simulink model "example_main_NDI_f16"  (R2020a)
settings: Solver=ode4  StartTime=0.0  StopTime=75  FixedStep=0.01  RelTol=1e-3
PreLoadFcn:
  | PreLoadFcn
values from neighbouring files (symbols this model uses):
  g = 32.17    [PreLoadFcn.m]
  N = [ 1      0     0.25 ... (first row only)    [PreLoadFcn.m]
  state0 = [IC.npos IC.epos IC.alt IC.q0 IC.q1 IC.q2 IC.q3  IC.p IC.q IC.r IC.alpha IC.beta IC.mu IC.Vt IC.chi IC.gamma]    [PreLoadFcn.m]
undefined symbols (not defined in the file or in its folder): Aactuator, ac, AeroCoeff, EngineTable, ft, IC, kg, m, Newton, PIController, Raphson, s, sigbuilder_block, slug
libraries: aerolibconvert2 x19, simulink x13, sharedutil x1
(part 3 of 6)

== system example_main_NDI_f16/F-16 Vehicle Systems Model/Vehicle/Actuators (no roll off)1 ==
  note: 這種建模方式會得到跟順淵不同的結果
  Command : Inport
  "Mach " : Inport  Port=2
  alt : Inport  Port=3
  alpha,beta : Inport  Port=4
  Aileron Saturation : Saturate  UpperLimit=21.5  LowerLimit=-21.5
  Demux1 : Demux  Outputs=6
  Elevator Saturation : Saturate  UpperLimit=25  LowerLimit=-25
  Engine block : Subsystem
  Fcn : Fcn  Expr=u(1)*cos(u(2))*cos(u(3))
  Integrator (degrees) : Integrator  Commented=through  InitialCondition=0.015206  UpperSaturationLimit=30  LowerSaturationLimit=-30
  Integrator (degrees)1 : Integrator  Commented=through  UpperSaturationLimit=30  LowerSaturationLimit=-30
  Integrator (degrees)2 : Integrator  Commented=on  UpperSaturationLimit=30  LowerSaturationLimit=-30
  Integrator(degrees) : Integrator  Commented=on  InitialCondition=-0.051516  UpperSaturationLimit=21.5  LowerSaturationLimit=-21.5
  "Integrator(degrees) " : Integrator  Commented=on  InitialCondition=-4.2454  UpperSaturationLimit=25  LowerSaturationLimit=-25
  Mux1 : Mux  Inputs=2
  Mux9 : Mux  Inputs=6
  Rate Limiter : RateLimiter  RisingSlewLimit=+60  FallingSlewLimit=-60  SampleTimeMode=inherited
  Rate Limiter1 : RateLimiter  RisingSlewLimit=+80  FallingSlewLimit=-80  SampleTimeMode=inherited
  Rate Limiter2 : RateLimiter  RisingSlewLimit=+120  FallingSlewLimit=-120  SampleTimeMode=inherited
  Rate Limiter3 : RateLimiter  RisingSlewLimit=+60  FallingSlewLimit=-60  SampleTimeMode=inherited
  Rate Limiter4 : RateLimiter  RisingSlewLimit=+60  FallingSlewLimit=-60  SampleTimeMode=inherited
  Rudder Saturation : Saturate  UpperLimit=30  LowerLimit=-30
  Saturation : Saturate  UpperLimit=50000  LowerLimit=0
  Saturation Dynamic : simulink/Discontinuities/Saturation Dynamic  OutMin=[]  OutMax=[]  OutDataTypeStr=Inherit: Same as second input  OutDataType=fixdt(1, 16)  OutScaling=2^-10  DoSatur=off
  TVC_Y Saturation : Saturate  UpperLimit=15  LowerLimit=-15
  TVC_Z Saturation : Saturate  UpperLimit=15  LowerLimit=-15
  Transfer Fcn{,1..4} (5 alike) : TransferFcn  Numerator=[20.202]  Denominator=[1 20.202]
  r2d2 : Gain  Gain=-1  SaturateOnIntegerOverflow=on  OutDataTypeStr=Inherit: Same as input  ParamDataTypeStr=Inherit: Same as input
  Actuator : Outport  VectorParamsAs1DForOutWhenUnconnected=off
  wires:
  Mux9/1 -> Actuator/1
  Command/1 -> Demux1/1
  Transfer Fcn/1 -> Mux9/2  "elevator"
  Transfer Fcn1/1 -> Mux9/3  "Aileron"
  Transfer Fcn2/1 -> Mux9/4  "Rudder"
  Saturation Dynamic/1 -> Mux9/1  "thrust"
  Transfer Fcn4/1 -> Mux9/6  "yaw vector"
  Transfer Fcn3/1 -> Mux9/5  "pitch vector"
  r2d2/1 -> Saturation/1
  alt/1 -> r2d2/1
  Demux1/1 -> Saturation Dynamic/2
  "Mach "/1 -> Mux1/1
  alpha,beta/1 -> Mux1/2
  Mux1/1 -> Fcn/1
  Fcn/1 -> Engine block/1(Mach)
  Saturation/1 -> Engine block/2(Attitude)
  Engine block/2(T_min) -> Saturation Dynamic/3
  Engine block/1(T_max) -> Saturation Dynamic/1
  Demux1/2 -> Elevator Saturation/1
  Elevator Saturation/1 -> Rate Limiter/1
  Demux1/3 -> Aileron Saturation/1
  Aileron Saturation/1 -> Rate Limiter1/1
  Demux1/4 -> Rudder Saturation/1
  Rudder Saturation/1 -> Rate Limiter2/1
  Demux1/5 -> TVC_Z Saturation/1
  TVC_Z Saturation/1 -> Rate Limiter3/1
  Demux1/6 -> TVC_Y Saturation/1
  TVC_Y Saturation/1 -> Rate Limiter4/1
  Rate Limiter/1 -> Transfer Fcn/1
  Rate Limiter1/1 -> Transfer Fcn1/1
  Rate Limiter2/1 -> Transfer Fcn2/1
  Rate Limiter3/1 -> Transfer Fcn3/1
  Rate Limiter4/1 -> Transfer Fcn4/1

== system example_main_NDI_f16/F-16 Vehicle Systems Model/Vehicle/Aerodynamics ==
  note: TODO: 這全部源自PlantData(物理系統)，不用感測器
  note: TODO: 這攻角、速度 來自感測器、AeroData System
  note: X
      | Y
      | Z
      | L
      | M
      | N
  note: 攻角 $\alpha$ 限制 -20 ~ 90度
      | 側滑角 $\beta$ 限制 -30 ~ 30 度
      | 馬赫數限制 0.1 ~ 0.6 度
  In Bus Element7 : Inport  PortName=EnvData  Element=P
  In Bus Element8 : Inport  PortName=EnvData  Element=AirDensity
  In Bus Element9 : Inport  PortName=EnvData  Element=qbar
  fcs_cmd : Inport  Port=2
  " SB (deg)" : Inport  Port=3
  In Bus Element : Inport  Port=4  PortName=PlantData  Element=p
  In Bus Element1 : Inport  Port=4  PortName=PlantData  Element=q
  In Bus Element2 : Inport  Port=4  PortName=PlantData  Element=r
  In Bus Element3 : Inport  Port=4  PortName=PlantData  Element=alpha
  In Bus Element10 : Inport  Port=4  PortName=PlantData  Element=alpha
  In Bus Element4 : Inport  Port=4  PortName=PlantData  Element=beta
  In Bus Element6 : Inport  Port=4  PortName=PlantData  Element=Vt
  In Bus Element5 : Inport  Port=4  PortName=PlantData  Element=Vt
  Aerofynamic Coefficients : Subsystem
  AirframeActuators (no roll off) : Subsystem
  Angle Conversion1 : aerolibconvert2/Angle Conversion  IU=rad  OU=deg
  Angle Conversion2 : aerolibconvert2/Angle Conversion  IU=rad  OU=deg
  Angle Conversion3 : aerolibconvert2/Angle Conversion  IU=rad  OU=deg
  Bus Creator : BusCreator  Inputs=4
  Bus Selector : BusSelector  OutputSignals=Elevator_deg,Aileron_deg,Rudder_deg
  Bus Selector1 : BusSelector  OutputSignals=Aileron_deg,Rudder_deg,Elevator_deg
  Bus Selector2 : BusSelector  OutputSignals=LEF_deg
  Cbar(ft)1 : Constant  Value=ac.cbar
  Ground : Ground
  Leading Edge Flap : Subsystem
  Mux1 : Mux  Inputs=3
  Mux2 : Mux
  Product{6,9..14} (7 alike) : Product
  Sref(ft^2) : Constant  Value=ac.S
  Velocity Conversion : aerolibconvert2/Velocity Conversion  IU=ft/s  OU=m/s
  b(ft)1 : Constant  Value=ac.b
  FM : Outport
  Bus Element Out : Outport  Port=2  PortName=ActSensor_Out
  wires:
  Bus Selector/2 -> Aerofynamic Coefficients/5(alieron (deg))  "<Aileron_deg>"
  " SB (deg)"/1 -> Aerofynamic Coefficients/7(SB (deg))
  In Bus Element1/1 -> Aerofynamic Coefficients/10(q)
  In Bus Element/1 -> Aerofynamic Coefficients/9(p)
  Bus Selector/3 -> Aerofynamic Coefficients/6(rudder (deg))  "<Rudder_deg>"
  Angle Conversion2/1 -> Aerofynamic Coefficients/2(beta (deg))
  Angle Conversion1/1 -> Aerofynamic Coefficients/1(alpha (deg))
  In Bus Element2/1 -> Aerofynamic Coefficients/11(r)
  [LEF_deg] -> Aerofynamic Coefficients/3(LEF (deg))
  Bus Selector/1 -> Aerofynamic Coefficients/4(elevator (deg))  "<Elevator_deg>"
  Ground/1 -> Aerofynamic Coefficients/13(h_AGL), Aerofynamic Coefficients/12(GearAngle)
  Mux1/1 -> Product9/2
  [qbar_S] -> Product9/1
  Aerofynamic Coefficients/6(Cn_T) -> Product14/2
  Aerofynamic Coefficients/5(Cm_T) -> Product12/2
  [qbar_S_cbar] -> Product12/1  "qbar_S_cbar"
  Aerofynamic Coefficients/4(Cl_T) -> Product13/2
  [qbar_S_b] -> Product13/1, Product14/1  "qbar_S_b"
  Aerofynamic Coefficients/1(CX_T) -> Mux1/1
  Aerofynamic Coefficients/2(CY_T) -> Mux1/2
  Aerofynamic Coefficients/3(CZ_T) -> Mux1/3
  Product13/1 -> Mux2/2
  Product12/1 -> Mux2/3
  Product14/1 -> Mux2/4
  Product9/1 -> Mux2/1
  Mux2/1 -> FM/1
  Sref(ft^2)/1 -> Product6/2
  b(ft)1/1 -> Product11/2  "b"
  Product11/1 -> [qbar_S_b]
  Product10/1 -> [qbar_S_cbar]
  Cbar(ft)1/1 -> Product10/2  "cbar"
  In Bus Element9/1 -> Product6/1  "qbar"
  Product6/1 -> Product11/1, Product10/1, [qbar_S]  "qbar_S"
  Leading Edge Flap/2(ActPositions) -> [LEF_deg]
  Velocity Conversion/1 -> Leading Edge Flap/1(vt (m/s))  "vt (m/s)"
  In Bus Element6/1 -> Aerofynamic Coefficients/8(vt (ft/s))
  In Bus Element8/1 -> Leading Edge Flap/2(rho (kg/m^3))
  In Bus Element7/1 -> Leading Edge Flap/3(P (Pa))
  AirframeActuators (no roll off)/1(ActPositions) -> Bus Selector/1
  fcs_cmd/1 -> AirframeActuators (no roll off)/1(fcs_cmd)
  In Bus Element3/1 -> Angle Conversion1/1
  In Bus Element4/1 -> Angle Conversion2/1
  In Bus Element5/1 -> Velocity Conversion/1  "vt (ft/s)"
  AirframeActuators (no roll off)/2(ActSensor_Out) -> Bus Selector1/1
  Bus Selector1/1 -> Bus Creator/1  "<Aileron_deg>"
  Bus Selector1/2 -> Bus Creator/2  "<Rudder_deg>"
  Bus Selector1/3 -> Bus Creator/3  "<Elevator_deg>"
  Bus Creator/1 -> Bus Element Out/1
  In Bus Element10/1 -> Angle Conversion3/1
  Angle Conversion3/1 -> Leading Edge Flap/4(alpha (deg))
  Leading Edge Flap/1(ActSensor_Out) -> Bus Selector2/1
  Bus Selector2/1 -> Bus Creator/4  "<LEF_deg>"

== system example_main_NDI_f16/F-16 Vehicle Systems Model/Vehicle/Propulsion ==
  note: 高度限制 0 ~ 50000 ft
      | 馬赫數限制 0 ~ 1 馬赫
  note: Thrust Vector Nozzle Module 向量噴嘴模組
  note: Commands_TVC_Z_pitch
      | Commands_TVC_Y_yaw
  note: Inlet 進氣道
  In Bus Element1 : Inport  PortName=EnvData  Element=Mach
  Bus Element In2 : Inport  Port=2  PortName=fadec_cmd
  In Bus Element2 : Inport  Port=2  PortName=fadec_cmd  Element=thrust
  Bus Element In1 : Inport  Port=3  PortName=PlantData  Element=beta
  Bus Element In : Inport  Port=3  PortName=PlantData  Element=alpha
  In Bus Element : Inport  Port=3  PortName=PlantData  Element=altitude
  Actuators : Subsystem
  Afterburning Turbofan Jet Engine : Subsystem
  Cos : Trigonometry  Operator=cos
  Cos1 : Trigonometry  Operator=cos
  Product : Product  Inputs=3
  Saturation Dynamic : simulink/Discontinuities/Saturation Dynamic  OutMin=[]  OutMax=[]  OutDataTypeStr=Inherit: Same as second input  OutDataType=fixdt(1, 16)  OutScaling=2^-10  DoSatur=off
  Thrust Vector Nozzle ZY : Subsystem
  nozzle position : Constant  Value=ac.lt
  r2d1 : Gain  Gain=-1  SaturateOnIntegerOverflow=on  OutDataTypeStr=Inherit: Same as input  ParamDataTypeStr=Inherit: Same as input
  FM : Outport
  Bus Element Out : Outport  Port=2  PortName=ActSensor_Out
  Bus Element Out1 : Outport  Port=3  PortName=PropData  Element=Tx
  Bus Element Out2 : Outport  Port=3  PortName=PropData  Element=Ty
  Bus Element Out3 : Outport  Port=3  PortName=PropData  Element=Tz
  Bus Element Out4 : Outport  Port=3  PortName=PropData  Element=T
  wires:
  Actuators/2(ActSensor_Out) -> Bus Element Out/1
  nozzle position/1 -> Thrust Vector Nozzle ZY/3(" lt")
  Actuators/1(ActPositions) -> Thrust Vector Nozzle ZY/2(Actuator (deg))
  Thrust Vector Nozzle ZY/1(FM) -> FM/1
  Product/1 -> Afterburning Turbofan Jet Engine/1(Mach)
  r2d1/1 -> Afterburning Turbofan Jet Engine/2(H (ft))
  Cos/1 -> Product/2
  Saturation Dynamic/1 -> Bus Element Out4/1, Thrust Vector Nozzle ZY/1(T)  "Thrust (lbf)"
  Bus Element In1/1 -> Cos1/1  "beta (rad)"
  Afterburning Turbofan Jet Engine/2(T_min) -> Saturation Dynamic/3
  In Bus Element1/1 -> Product/1
  Cos1/1 -> Product/3
  Bus Element In/1 -> Cos/1  "alpha (rad)"
  Afterburning Turbofan Jet Engine/1(T_max) -> Saturation Dynamic/1
  In Bus Element/1 -> r2d1/1
  In Bus Element2/1 -> Saturation Dynamic/2  "Commands_Tc"
  Bus Element In2/1 -> Actuators/1(Commands)
  Thrust Vector Nozzle ZY/2(Tx) -> Bus Element Out1/1
  Thrust Vector Nozzle ZY/3(Ty) -> Bus Element Out2/1
  Thrust Vector Nozzle ZY/4(Tz) -> Bus Element Out3/1

== system example_main_NDI_f16/F-16 Vehicle Systems Model/pqr NDI Controller/TVC OFF ==
  note: 【無向量噴嘴控制】
      | (註：有/無向量噴嘴的差異之處在於 "粉紅色模塊" 的內容)
  note: 沒有控制配置，也不需要，
      | 因為沒有多餘的控制面可用
  note: gp_da1
      | gp_da2
      | gp_dr1
      | gp_dr2
      | m_de
      | gr_da1
      | gr_da2
      | gr_dr1
      | gr_dr2
  note: $\hat{L}, \hat{M}, \hat{N}$
  coef M : Inport
  control g : Inport  Port=2
  pqr dot desire : Inport  Port=3
  In Bus Element : Inport  Port=4  PortName=PlantData  Element=PropBus.T
  p q r : Inport  Port=5
  In Bus Element2 : Inport  Port=6  PortName=AirData  Element=alpha
  In Bus Element1 : Inport  Port=6  PortName=AirData  Element=Vt
  " f1" : MATLAB Function  TreatAsAtomicUnit=on
  Constant : Constant  Value=0
  Constant1 : Constant  Value=0
  Ix(slug*ft^2)1 : Constant  Value=ac.Ix
  Ixz(slug*ft^2)1 : Constant  Value=ac.Ixz
  Iy(slug*ft^2)1 : Constant  Value=ac.Iy
  Iz(slug*ft^2)1 : Constant  Value=ac.Iz
  Sum : Sum  Inputs=+-|
  Terminator : Terminator
  Terminator1 : Terminator
  control matrix g1 : Subsystem
  innear NDI : MATLAB Function  TreatAsAtomicUnit=on
  TVC_z : Outport  VectorParamsAs1DForOutWhenUnconnected=off
  "TVC_y " : Outport  Port=2  VectorParamsAs1DForOutWhenUnconnected=off
  elevator : Outport  Port=3  VectorParamsAs1DForOutWhenUnconnected=off
  aileron : Outport  Port=4  VectorParamsAs1DForOutWhenUnconnected=off
  rudder : Outport  Port=5  VectorParamsAs1DForOutWhenUnconnected=off
  wires:
  Iy(slug*ft^2)1/1 -> " f1"/4(Iy)
  Ixz(slug*ft^2)1/1 -> " f1"/6(Ixz)
  Iz(slug*ft^2)1/1 -> " f1"/5(Iz)
  pqr dot desire/1 -> Sum/1
  Sum/1 -> innear NDI/1(y_bar)
  p q r/1 -> " f1"/2(pqr)
  Ix(slug*ft^2)1/1 -> " f1"/3(Ix)
  " f1"/1(f) -> Sum/2
  Constant1/1 -> "TVC_y "/1
  control matrix g1/1(g_1 Row1) -> innear NDI/2(g_row1)
  innear NDI/3(rudder) -> rudder/1
  control matrix g1/3(g_1 Row3) -> innear NDI/4(g_row3)
  innear NDI/2(elevator) -> elevator/1
  control g/1 -> control matrix g1/1(coef g)
  In Bus Element/1 -> control matrix g1/2(Thrust T)
  innear NDI/1(aileron) -> aileron/1
  control matrix g1/2(g_1 Row2) -> innear NDI/3(g_row2)
  coef M/1 -> " f1"/1(moments)
  Constant/1 -> TVC_z/1
  In Bus Element1/1 -> Terminator/1
  In Bus Element2/1 -> Terminator1/1

== system example_main_NDI_f16/F-16 Vehicle Systems Model/pqr NDI Controller/TVC ON ==
  note: $\hat{L}, \hat{M}, \hat{N}$
  note: TODO:
      | 1. 控制配置的權重矩陣 參數化、拿出來外面、放進PreLoadFcn.m
      | 2. 改成Variant Subsystem
  note: 控制配置：
      | 1. 菊鍊式
      | 2. 聯動式
  note: gp_da1
      | gp_da2
      | gp_dr1
      | gp_dr2
      | m_de
      | gr_da1
      | gr_da2
      | gr_dr1
      | gr_dr2
  note: 【有向量噴嘴控制】
      | (註：有/無向量噴嘴的差異之處在於 "粉紅色模塊" 的內容)
  coef M : Inport
  control g : Inport  Port=2
  pqr dot desire : Inport  Port=3
  In Bus Element : Inport  Port=4  PortName=PlantData  Element=PropBus.T
  In Bus Element2 : Inport  Port=5  PortName=AirData  Element=alpha
  In Bus Element1 : Inport  Port=5  PortName=AirData  Element=Vt
  p q r : Inport  Port=6
  " f1" : MATLAB Function  TreatAsAtomicUnit=on
  Control Allocation : MATLAB Function  TreatAsAtomicUnit=on
  Ix(slug*ft^2)1 : Constant  Value=ac.Ix
  Ixz(slug*ft^2)1 : Constant  Value=ac.Ixz
  Iy(slug*ft^2)1 : Constant  Value=ac.Iy
  Iz(slug*ft^2)1 : Constant  Value=ac.Iz
  Sum : Sum  Inputs=+-|
  control matrix g1 : Subsystem
  weighting matrix N : Constant  Value=N
  TVC_z : Outport  VectorParamsAs1DForOutWhenUnconnected=off
  "TVC_y " : Outport  Port=2  VectorParamsAs1DForOutWhenUnconnected=off
  elevator : Outport  Port=3  VectorParamsAs1DForOutWhenUnconnected=off
  aileron : Outport  Port=4  VectorParamsAs1DForOutWhenUnconnected=off
  rudder : Outport  Port=5  VectorParamsAs1DForOutWhenUnconnected=off
  wires:
  coef M/1 -> " f1"/1(moments)
  p q r/1 -> " f1"/2(pqr)
  " f1"/1(f) -> Sum/2
  Sum/1 -> Control Allocation/1(y_bar)
  pqr dot desire/1 -> Sum/1
  In Bus Element/1 -> control matrix g1/2(Thrust T)
  control g/1 -> control matrix g1/1(coef g)
  control matrix g1/1(g_1 Row1) -> Control Allocation/2(g_row1)
  control matrix g1/2(g_1 Row2) -> Control Allocation/3(g_row2)
  control matrix g1/3(g_1 Row3) -> Control Allocation/4(g_row3)
  Control Allocation/3(rudder) -> rudder/1
  Control Allocation/2(elevator) -> elevator/1
  Control Allocation/1(aileron) -> aileron/1
  Control Allocation/4(TVC_y) -> "TVC_y "/1
  Control Allocation/5(TVC_z) -> TVC_z/1
  In Bus Element2/1 -> Control Allocation/6(alpha)
  Iy(slug*ft^2)1/1 -> " f1"/4(Iy)
  Ix(slug*ft^2)1/1 -> " f1"/3(Ix)
  Iz(slug*ft^2)1/1 -> " f1"/5(Iz)
  Ixz(slug*ft^2)1/1 -> " f1"/6(Ixz)
  weighting matrix N/1 -> Control Allocation/7(N)
  In Bus Element1/1 -> Control Allocation/5(Vt)

== system example_main_NDI_f16/F-16 Vehicle Systems Model/μαβ NDI Controller/command matrix (5.5.4) ==
  note: $g_2 {\left(x\right)}={\left[\begin{array}{ccc} g_{\mu_p } & g_{\mu_q } & g_{\mu_r } \\ g_{\alpha_p } & g_{\alpha_q } & g_{\alpha_r } \\ g_{\beta_p } & g_{\beta_q } & g_{\beta_r } \end{array}\right]}={\left[\begin{array}{ccc} \mathrm{cos}\alpha \mathrm{sec}\beta & 0 & \mathrm{sin}\alpha \mathrm{sec}\beta \\ -\mathrm{cos}\alpha \mathrm{tan}\beta & 1 & -\mathrm{sin}\alpha \mathrm{tan}\beta \\ \mathrm{sin}\alpha & 0 & -\mathrm{cos}\alpha \end{array}\right]}$
  α : Inport
  β : Inport  Port=2
  (1,1) : Fcn  Expr=1/cos(u(2)) * cos(u(1))
  (1,2) : Constant  Value=0
  (1,3) : Fcn  Expr=1/cos(u(2)) * sin(u(1))
  (2,1) : Fcn  Expr=-tan(u(2)) * cos(u(1))
  (2,2) : Constant
  (2,3) : Fcn  Expr=-tan(u(2)) * sin(u(1))
  (3,1) : Fcn  Expr=sin(u(1))
  (3,2) : Constant  Value=0
  (3,3) : Fcn  Expr=-cos(u(1))
  Create 3x3 Matrix : sharedutil/Create 3x3 Matrix  aMode=aMode
      settings: SourceProductBaseCode=AE,PW,MT,VE,VP
  Mux4 : Mux  Inputs=2
  g2 : Outport  VectorParamsAs1DForOutWhenUnconnected=off
  wires:
  α/1 -> Mux4/1
  β/1 -> Mux4/2
  Mux4/1 -> (3,3)/1, (3,1)/1, (2,3)/1, (1,1)/1, (1,3)/1, (2,1)/1
  Create 3x3 Matrix/1 -> g2/1
  (2,2)/1 -> Create 3x3 Matrix/5
  (2,1)/1 -> Create 3x3 Matrix/4
  (2,3)/1 -> Create 3x3 Matrix/6
  (1,3)/1 -> Create 3x3 Matrix/3
  (3,1)/1 -> Create 3x3 Matrix/7
  (1,2)/1 -> Create 3x3 Matrix/2
  (3,2)/1 -> Create 3x3 Matrix/8
  (1,1)/1 -> Create 3x3 Matrix/1
  (3,3)/1 -> Create 3x3 Matrix/9

== system example_main_NDI_f16/F-16 Vehicle Systems Model/μαβ NDI Controller/f2 (5.5.3) ==
  note: 有指定port dimensions=3。
      | 否則，雖然可以正常執行程式，
      | 但是t=0會跳出錯誤訊息說下一模塊"attitude NDI"內的矩陣運算的dimensions不一致
  note: mu alpha beta
  note: 11 gravity
  note: 10 T
  note: 9 mass
  note: 8 L
  note: 7 Y
  note: 6 D
  note: 1 Vt alpha beta mu gamma
  note: 11 gravity
  note: 9 mass
  note: 6 Xbar Ybar Zbar
  note: 1 Vinf alpha beta mu gamma
  note: 10 T
  aero V : Inport
  X,Y,Z : Inport  Port=2
  gravity : Inport  Port=3
  Thrust : Inport  Port=4
  Add : Sum  Inputs=+++
  Drag : Fcn  Expr=-u(6)*cos(u(2))*cos(u(3))-u(7)*sin( u(3) )-u(8)*sin(u(2))*cos(u(3))
  Lift : Fcn  Expr=u(6)*sin(u(2))-u(8)*cos(u(2))
  Mux : Mux  Inputs=3
  Mux1 : Mux  Inputs=7
  Mux2 : Mux  Inputs=2
  Side Force : Fcn  Expr=-u(6)*cos(u(2))*sin(u(3))+u(7)*cos( u(3) )-u(8)*sin(u(2))*sin(u(3))
  f_alpha : Fcn  Expr=( -u(8)+u(9)*u(11)*cos(u(5))*cos(u(4))-u(10)*sin(u(2)) ) / ( u(9)*u(1)*cos(u(3)) )
  f_beta : Fcn  Expr=( u(7)*cos(u(3))+u(9)*u(11)*cos(u(5))*sin(u(4))-u(10)*cos(u(2))*sin(u(3)) ) / ( u(9)*u(1) )
  f_mu1 : Fcn  Expr=u(8)*( tan(u(5))*sin(u(4))+tan(u(3)) ) / ( u(9)*u(1) )
  f_mu2 : Fcn  Expr=(u(7)*tan(u(5))*cos(u(4))*cos(u(3)) -u(9)*u(11)*cos(u(5))*cos(u(4))*tan(u(3)) ) / ( u(9)*u(1) )
  f_mu3 : Fcn  Expr=u(10)*( sin(u(2))*tan(u(5))*sin(u(4)) + sin(u(2))*tan(u(3)) - cos(u(2))*tan(u(5))*cos(u(4))*sin(u(3)) ) / ( u(9)*u(1) )
  m(slugs) : Constant  Value=ac.m
  f2 : Outport  PortDimensions=3  VectorParamsAs1DForOutWhenUnconnected=off
  D : Outport  Port=2  VectorParamsAs1DForOutWhenUnconnected=off
  Y : Outport  Port=3  VectorParamsAs1DForOutWhenUnconnected=off
  L : Outport  Port=4  VectorParamsAs1DForOutWhenUnconnected=off
  wires:
  Mux/1 -> f2/1
  f_beta/1 -> Mux/3
  aero V/1 -> Mux1/1, Mux2/1  "Vt, α, β, μ, γ"
  X,Y,Z/1 -> Mux2/2  "Xbar, Ybar, Zbar"
  Mux2/1 -> Lift/1, Drag/1, Side Force/1
  Mux1/1 -> f_alpha/1, f_beta/1, f_mu2/1, f_mu1/1, f_mu3/1
  Drag/1 -> Mux1/2, D/1  "D"
  Side Force/1 -> Mux1/3, Y/1  "Y"
  Lift/1 -> Mux1/4, L/1  "L"
  m(slugs)/1 -> Mux1/5
  Thrust/1 -> Mux1/6  "T"
  gravity/1 -> Mux1/7  "g"
  f_alpha/1 -> Mux/2
  f_mu2/1 -> Add/2
  f_mu1/1 -> Add/1
  Add/1 -> Mux/1
  f_mu3/1 -> Add/3

== system example_main_NDI_f16/F-16 Vehicle Systems Model/Aerodynamic1/NDI Aerofynamic Coefficients/CXT ==
  note: 氣動力表格僅提供到攻角到
      | 45度，超過45度後皆採用45
      | 度的氣動力係數
  note: $\Delta C_{X_{LEF} } =C_{X_{LEF} } {\left(\alpha ,\beta \right)}-C_X {\left(\alpha ,\beta ,\delta_e =0°\right)}$
  note: $C_{X,T} =C_X {\left(\alpha ,\beta ,\delta_e \right)}+\Delta C_{X_{LEF} } ∙{\left(1-\frac{\delta_{LEF} }{25°}\right)}+\frac{q\bar{c} }{2V_T }∙{\left[C_{X_q } {\left(\alpha \right)}+\Delta C_{X_{q_{LEF} } } {\left(\alpha \right)}∙{\left(1-\frac{\delta_{LEF} }{25°}\right)}\right]}+\Delta C_{X_{SB} } {\left(\alpha \right)}∙{\left(\frac{\delta_{SB} }{60°}\right)}$
  note: 體軸 x 方向之氣動力係數 (total x-axis force coefficient)：
  alpha (deg) : Inport
  beta (deg) : Inport  Port=2
  elevator (deg) : Inport  Port=3
  dlef : Inport  Port=4
  qc_2v : Inport  Port=5
  sb : Inport  Port=6
  Add : Sum  Inputs=+-
  Add1 : Sum  Inputs=++++
  Add2 : Sum
  Cx : Interpolation_n-D  NumberOfTableDimensions=3  Table=AeroCoeff.Cx
      settings: InputPortMap=u0,u1,u2,u3,u4,u5
  Cx_elevator0 : Interpolation_n-D  Table=AeroCoeff.Cx_elevator0
  Cx_lef : Interpolation_n-D  Table=AeroCoeff.Cx_lef
  Cx_q : Interpolation_n-D  NumberOfTableDimensions=1  Table=AeroCoeff.Cx_q
      settings: InputPortMap=u0,u1
  Cx_q_lef : Interpolation_n-D  NumberOfTableDimensions=1  Table=AeroCoeff.Cx_q_lef
      settings: InputPortMap=u0,u1
  Product{,1..3} (4 alike) : Product
  alpha Prelookup : PreLookup  BreakpointsData=AeroCoeff.alpha_prelookup  IndexSearchMethod=Linear search  BeginIndexSearchUsingPreviousIndexResult=on  DiagnosticForOutOfRangeInput=Warning
  beta Prelookup : PreLookup  BreakpointsData=AeroCoeff.beta_prelookup  IndexSearchMethod=Linear search  BeginIndexSearchUsingPreviousIndexResult=on  DiagnosticForOutOfRangeInput=Warning
  dCX_sb : Interpolation_n-D  NumberOfTableDimensions=1  Table=AeroCoeff.dCX_sb
      settings: InputPortMap=u0,u1
  elevator Prelookup : PreLookup  BreakpointsData=AeroCoeff.elevator_prelookup2  IndexSearchMethod=Linear search  BeginIndexSearchUsingPreviousIndexResult=on  DiagnosticForOutOfRangeInput=Warning
  Cx_tot : Outport  VectorParamsAs1DForOutWhenUnconnected=off
  wires:
  beta Prelookup/2 -> Cx_elevator0/4, Cx_lef/4, Cx/4
  alpha (deg)/1 -> alpha Prelookup/1
  beta Prelookup/1 -> Cx_elevator0/3, Cx_lef/3, Cx/3
  Cx_lef/1 -> Add/1
  alpha Prelookup/1 -> Cx_q_lef/1, dCX_sb/1, Cx_q/1, Cx_elevator0/1, Cx/1, Cx_lef/1
  elevator Prelookup/2 -> Cx/6
  elevator (deg)/1 -> elevator Prelookup/1
  beta (deg)/1 -> beta Prelookup/1
  Add/1 -> Product/1
  alpha Prelookup/2 -> Cx_q_lef/2, dCX_sb/2, Cx_q/2, Cx_elevator0/2, Cx_lef/2, Cx/2
  Product/1 -> Add1/2
  elevator Prelookup/1 -> Cx/5
  Add2/1 -> Product2/1
  Cx/1 -> Add1/1
  Cx_elevator0/1 -> Add/2
  Cx_q_lef/1 -> Product1/1
  Product1/1 -> Add2/2
  Cx_q/1 -> Add2/1
  dlef/1 -> Product/2, Product1/2
  Product2/1 -> Add1/3
  Add1/1 -> Cx_tot/1
  qc_2v/1 -> Product2/2
  dCX_sb/1 -> Product3/1
  sb/1 -> Product3/2
  Product3/1 -> Add1/4

== system example_main_NDI_f16/F-16 Vehicle Systems Model/Aerodynamic1/NDI Aerofynamic Coefficients/CYT ==
  note: 氣動力表格僅提供到攻角到
      | 45度，超過45度後皆採用45
      | 度的氣動力係數
  note: 氣動力表格僅提供到攻角到
      | 45度，超過45度後皆採用45
      | 度的氣動力係數
  note: 體軸 y 方向之氣動力係數 (total y-axis force coefficient)：
  note: $\Delta C_{Y_{LEF} }=C_{Y_{LEF} } {\left(\alpha ,\beta \right)}\ \ -C_Y {\left(\alpha ,\beta \right)}$
  note: $\Delta C_{Y_{\delta_r } }=C_{Y_{\delta_r =30°} } {\left(\alpha ,\beta \right)}-C_Y {\left(\alpha ,\beta \right)}$
  note: $C_{Y,T} =C_Y {\left(\alpha ,\beta \right)}+\Delta C_{Y_{LEF} } ∙{\left(1-\frac{\delta_{LEF} }{25°}\right)}+\frac{pb}{2V_T }∙{\left[C_{Y_p } {\left(\alpha \right)}+\Delta C_{{Y_p }_{LEF} } {\left(\alpha \right)}∙{\left(1-\frac{\delta_{LEF} }{25°}\right)}\right]}+\frac{rb}{2V_T }∙{\left[C_{Y_r } {\left(\alpha \right)}+\Delta C_{{Y_r }_{LEF} } {\left(\alpha \right)}∙{\left(1-\frac{\delta_{LEF} }{25°}\right)}\right]}+{\left[\Delta C_{Y_{\delta_a } } +\Delta C_{Y_{{\delta_a }_{LEF} } } ∙{\left(1-\frac{\delta_{LEF} }{25°}\right)}\right]}∙{\left(\frac{\delta_a }{20°}\right)}+\Delta C_{Y_{\delta_r } } ∙{\left(\frac{\delta_r }{30°}\right)}$
  note: $\Delta C_{Y_{{\delta_a }_{LEF} } } =C_{Y_{{\delta_a =20°}_{LEF} } } {\left(\alpha ,\beta \right)}-C_{Y_{LEF} } {\left(\alpha ,\beta \right)}-\Delta C_{Y_{\delta_a } }$
  note: $\Delta C_{Y_{\delta_a } }=C_{Y_{\delta_a =20°} } {\left(\alpha ,\beta \right)}-C_Y {\left(\alpha ,\beta \right)}$
  alpha (deg) : Inport
  beta (deg) : Inport  Port=2
  dlef : Inport  Port=3
  dail : Inport  Port=4
  drud : Inport  Port=5
  rb_2v : Inport  Port=6
  pb_2v : Inport  Port=7
  Add : Sum  Inputs=-+
  Add1 : Sum  Inputs=-+
  Add2 : Sum  Inputs=+--
  Add3 : Sum  Inputs=+-
  Add4 : Sum  Inputs=++++++
  Add5 : Sum
  Add6 : Sum
  Add7 : Sum
  Add8 : Sum  Inputs=++++
  CY : Interpolation_n-D  Table=AeroCoeff.CY
  CY_delta_ail : Interpolation_n-D  Table=AeroCoeff.CY_delta_ail
  CY_delta_ail_lef : Interpolation_n-D  Table=AeroCoeff.CY_delta_ail_lef
  CY_delta_r : Interpolation_n-D  Table=AeroCoeff.CY_delta_r
  CY_lef : Interpolation_n-D  Table=AeroCoeff.CY_lef
  CY_p : Interpolation_n-D  NumberOfTableDimensions=1  Table=AeroCoeff.CY_p
      settings: InputPortMap=u0,u1
  CY_r : Interpolation_n-D  NumberOfTableDimensions=1  Table=AeroCoeff.CY_r
      settings: InputPortMap=u0,u1
  Product{,1..7} (8 alike) : Product
  alpha Prelookup : PreLookup  BreakpointsData=AeroCoeff.alpha_prelookup  IndexSearchMethod=Linear search  BeginIndexSearchUsingPreviousIndexResult=on  DiagnosticForOutOfRangeInput=Warning
  beta Prelookup : PreLookup  BreakpointsData=AeroCoeff.beta_prelookup  IndexSearchMethod=Linear search  BeginIndexSearchUsingPreviousIndexResult=on  DiagnosticForOutOfRangeInput=Warning
  dCY_p_lef : Interpolation_n-D  NumberOfTableDimensions=1  Table=AeroCoeff.dCY_p_lef
      settings: InputPortMap=u0,u1
  dCY_r_lef : Interpolation_n-D  NumberOfTableDimensions=1  Table=AeroCoeff.dCY_r_lef
      settings: InputPortMap=u0,u1
  Cy_tot : Outport  VectorParamsAs1DForOutWhenUnconnected=off
  Cy_tot_n_mom : Outport  Port=2  VectorParamsAs1DForOutWhenUnconnected=off
  Cy_tot_n_da : Outport  Port=3  VectorParamsAs1DForOutWhenUnconnected=off
  Cy_tot_n_dr : Outport  Port=4  VectorParamsAs1DForOutWhenUnconnected=off
  wires:
  Add3/1 -> Cy_tot_n_dr/1, Product3/1
  beta Prelookup/2 -> CY_delta_r/4, CY_delta_ail_lef/4, CY_delta_ail/4, CY/4, CY_lef/4
  beta Prelookup/1 -> CY_delta_r/3, CY_delta_ail_lef/3, CY_delta_ail/3, CY/3, CY_lef/3
  Product7/1 -> Add4/6, Add8/4
  dlef/1 -> Product1/2, Product/2, Product4/2, Product6/1
  alpha Prelookup/1 -> dCY_p_lef/1, CY_p/1, dCY_r_lef/1, CY_r/1, CY_delta_r/1, CY_delta_ail_lef/1, CY_delta_ail/1, CY_lef/1, CY/1
  Add4/1 -> Cy_tot/1
  Add5/1 -> Cy_tot_n_da/1, Product2/1
  CY_p/1 -> Add7/1
  Add1/1 -> Add2/3, Add5/1
  CY_lef/1 -> Add/2, Add2/2
  Add/1 -> Product/1
  dCY_p_lef/1 -> Product6/2
  CY_delta_r/1 -> Add3/1
  CY_delta_ail_lef/1 -> Add2/1
  dCY_r_lef/1 -> Product4/1
  alpha (deg)/1 -> alpha Prelookup/1
  CY_r/1 -> Add6/1
  Product4/1 -> Add6/2
  Add2/1 -> Product1/1
  Product3/1 -> Add4/4
  CY/1 -> Add8/1, Add4/1, Add/1, Add1/1, Add3/2
  Product2/1 -> Add4/3
  Product/1 -> Add4/2, Add8/2
  alpha Prelookup/2 -> CY_p/2, dCY_p_lef/2, dCY_r_lef/2, CY_r/2, CY_delta_r/2, CY_delta_ail_lef/2, CY_delta_ail/2, CY_lef/2, CY/2
  Product6/1 -> Add7/2
  Add6/1 -> Product5/2
  Add7/1 -> Product7/2
  Product5/1 -> Add4/5, Add8/3
  Product1/1 -> Add5/2
  CY_delta_ail/1 -> Add1/2
  beta (deg)/1 -> beta Prelookup/1
  dail/1 -> Product2/2
  drud/1 -> Product3/2
  pb_2v/1 -> Product7/1
  rb_2v/1 -> Product5/1
  Add8/1 -> Cy_tot_n_mom/1

== system example_main_NDI_f16/F-16 Vehicle Systems Model/Aerodynamic1/NDI Aerofynamic Coefficients/CZT ==
  note: CZ
  note: 氣動力表格僅提供到攻角到
      | 45度，超過45度後皆採用45
      | 度的氣動力係數
  note: $\Delta C_{Z_{LEF} } =C_{Z_{LEF} } {\left(\alpha ,\beta \right)}-C_Z {\left(\alpha ,\beta ,\delta_e =0°\right)}$
  note: $C_{Z,T} =C_Z {\left(\alpha ,\beta ,\delta_e \right)}+\Delta C_{Z_{LEF} } ∙{\left(1-\frac{\delta_{LEF} }{25°}\right)}+\frac{q\bar{c} }{2V_T }∙{\left[C_{Z_q } {\left(\alpha \right)}+\Delta C_{Z_{q_{LEF} } } {\left(\alpha \right)}∙{\left(1-\frac{\delta_{LEF} }{25°}\right)}\right]}+\ \Delta C_{Z_{SB} } {\left(\alpha \right)}∙{\left(\frac{\delta_{SB} }{60°}\right)}$
  note: 體軸 z 方向之氣動力係數 (total z-axis force coefficient)：
  alpha (deg) : Inport
  beta (deg) : Inport  Port=2
  elevator (deg) : Inport  Port=3
  dlef : Inport  Port=4
  qc_2v : Inport  Port=5
  sb : Inport  Port=6
  Add : Sum  Inputs=+-
  Add1 : Sum  Inputs=++++
  Add2 : Sum
  Add3 : Sum  Inputs=+++
  Add4 : Sum  Inputs=+++
  Bias : Bias  Bias=0.1
  Bias1 : Bias  Bias=-0.1
  CZ : Interpolation_n-D  NumberOfTableDimensions=3  Table=AeroCoeff.CZ
      settings: InputPortMap=u0,u1,u2,u3,u4,u5
  CZ_elevator0 : Interpolation_n-D  Table=AeroCoeff.CZ_elevator0
  CZ_lef : Interpolation_n-D  Table=AeroCoeff.CZ_lef
  CZ_q : Interpolation_n-D  NumberOfTableDimensions=1  Table=AeroCoeff.CZ_q
      settings: InputPortMap=u0,u1
  Product{,1..3} (4 alike) : Product
  alpha Prelookup : PreLookup  BreakpointsData=AeroCoeff.alpha_prelookup  IndexSearchMethod=Linear search  BeginIndexSearchUsingPreviousIndexResult=on  DiagnosticForOutOfRangeInput=Warning
  beta Prelookup : PreLookup  BreakpointsData=AeroCoeff.beta_prelookup  IndexSearchMethod=Linear search  BeginIndexSearchUsingPreviousIndexResult=on  DiagnosticForOutOfRangeInput=Warning
  dCZ_q_lef : Interpolation_n-D  NumberOfTableDimensions=1  Table=AeroCoeff.dCZ_q_lef
      settings: InputPortMap=u0,u1
  dCZ_sb : Interpolation_n-D  NumberOfTableDimensions=1  Table=AeroCoeff.dCZ_sb
      settings: InputPortMap=u0,u1
  elevator Prelookup : PreLookup  BreakpointsData=AeroCoeff.elevator_prelookup2  IndexSearchMethod=Linear search  BeginIndexSearchUsingPreviousIndexResult=on  DiagnosticForOutOfRangeInput=Warning
  elevator Prelookup1 : PreLookup  BreakpointsData=AeroCoeff.elevator_prelookup2  IndexSearchMethod=Linear search  BeginIndexSearchUsingPreviousIndexResult=on  DiagnosticForOutOfRangeInput=Warning
  elevator Prelookup2 : PreLookup  BreakpointsData=AeroCoeff.elevator_prelookup2  IndexSearchMethod=Linear search  BeginIndexSearchUsingPreviousIndexResult=on  DiagnosticForOutOfRangeInput=Warning
  same as CZ : Interpolation_n-D  NumberOfTableDimensions=3  Table=AeroCoeff.CZ
      settings: InputPortMap=u0,u1,u2,u3,u4,u5
  same_as_CZ : Interpolation_n-D  NumberOfTableDimensions=3  Table=AeroCoeff.CZ
      settings: InputPortMap=u0,u1,u2,u3,u4,u5
  Cz_tot : Outport  VectorParamsAs1DForOutWhenUnconnected=off
  Cz_tot_plus : Outport  Port=2  VectorParamsAs1DForOutWhenUnconnected=off
  Cz_tot_minus : Outport  Port=3  VectorParamsAs1DForOutWhenUnconnected=off
  wires:
  Product2/1 -> Add1/3, Add4/2, Add3/2
  alpha Prelookup/2 -> same as CZ/2, same_as_CZ/2, dCZ_sb/2, dCZ_q_lef/2, CZ_q/2, CZ_elevator0/2, CZ_lef/2, CZ/2
  Add1/1 -> Cz_tot/1
  elevator Prelookup/1 -> CZ/5
  CZ_q/1 -> Add2/1
  beta Prelookup/2 -> same as CZ/4, same_as_CZ/4, CZ_elevator0/4, CZ/4, CZ_lef/4
  CZ_lef/1 -> Add/1
  dCZ_q_lef/1 -> Product1/1
  Product1/1 -> Add2/2
  Add2/1 -> Product2/1
  CZ_elevator0/1 -> Add/2
  Add/1 -> Product/1
  dlef/1 -> Product1/2, Product/2
  Product/1 -> Add3/1, Add4/1, Add1/2
  CZ/1 -> Add1/1
  beta Prelookup/1 -> same as CZ/3, same_as_CZ/3, CZ_elevator0/3, CZ_lef/3, CZ/3
  alpha Prelookup/1 -> same as CZ/1, same_as_CZ/1, dCZ_sb/1, dCZ_q_lef/1, CZ_q/1, CZ_elevator0/1, CZ_lef/1, CZ/1
  alpha (deg)/1 -> alpha Prelookup/1
  elevator Prelookup/2 -> CZ/6
  qc_2v/1 -> Product2/2
  beta (deg)/1 -> beta Prelookup/1
  elevator (deg)/1 -> elevator Prelookup/1, Bias1/1, Bias/1
  Bias/1 -> elevator Prelookup1/1
  Bias1/1 -> elevator Prelookup2/1
  elevator Prelookup1/2 -> same_as_CZ/6
  elevator Prelookup1/1 -> same_as_CZ/5
  elevator Prelookup2/2 -> same as CZ/6
  elevator Prelookup2/1 -> same as CZ/5
  same_as_CZ/1 -> Add3/3
  same as CZ/1 -> Add4/3
  Add3/1 -> Cz_tot_plus/1
  Add4/1 -> Cz_tot_minus/1
  sb/1 -> Product3/2
  dCZ_sb/1 -> Product3/1
  Product3/1 -> Add1/4

== system example_main_NDI_f16/F-16 Vehicle Systems Model/Aerodynamic1/NDI Aerofynamic Coefficients/ClT ==
  note: 氣動力表格僅提供到攻角到
      | 45度，超過45度後皆採用45
      | 度的氣動力係數
  note: 氣動力表格僅提供到攻角到
      | 45度，超過45度後皆採用45
      | 度的氣動力係數
  note: $\Delta C_{l_{LEF} } =C_{l_{LEF} } {\left(\alpha ,\beta \right)}-C_l {\left(\alpha ,\beta ,\delta_e =0°\right)}$
  note: $\Delta C_{l_{\delta_a } } =C_{l_{\delta_a =20°} } {\left(\alpha ,\beta \right)}-C_l {\left(\alpha ,\beta ,\delta_e =0°\right)}$
  note: $C_{l,T} =C_l {\left(\alpha ,\beta ,\delta_e \right)}+\Delta C_{l_{LEF} } ∙{\left(1-\frac{\delta_{LEF} }{25°}\right)}+\frac{pb}{2V_T }∙{\left[C_{l_p } {\left(\alpha \right)}+\Delta C_{l_{p_{LEF} } } {\left(\alpha \right)}∙{\left(1-\frac{\delta_{LEF} }{25°}\right)}+\frac{rb}{2V_T }∙{\left[C_{l_r } {\left(\alpha \right)}+\Delta C_{l_{r_{LEF} } } {\left(\alpha \right)}∙{\left(1-\frac{\delta_{LEF} }{25°}\right)}\right]}+\Delta C_{l_{\beta } } {\left(\alpha \right)}∙\beta +{\left[\Delta C_{l_{\delta_a } } +\Delta C_{l_{{\delta_a }_{LEF} } } ∙{\left(1-\frac{\delta_{LEF} }{25°}\right)}\right]}∙{\left(\frac{\delta_a }{20°}\right)}+\Delta C_{l_{\delta_r } } ∙{\left(\frac{\delta_r }{30°}\right)}\right]}$
  note: 側滾氣動力矩係數 (total rolling moment coefficient)：
  note: $\Delta C_{l_{\delta_r } } =C_{l_{\delta_r =30°} } {\left(\alpha ,\beta \right)}-C_l {\left(\alpha ,\beta ,\delta_e =0°\right)}$
  note: $\Delta C_{l_{{\delta_a }_{LEF} } } =C_{l_{{\delta_a =20°}_{LEF} } } {\left(\alpha ,\beta \right)}-C_{l_{LEF} } {\left(\alpha ,\beta \right)}-\Delta C_{l_{\delta_a } }$
  alpha (deg) : Inport
  beta (deg) : Inport  Port=2
  elevator (deg) : Inport  Port=3
  dlef : Inport  Port=4
  rb_2v : Inport  Port=5
  pb_2v : Inport  Port=6
  Cl : Interpolation_n-D  NumberOfTableDimensions=3  Table=AeroCoeff.Cl
      settings: InputPortMap=u0,u1,u2,u3,u4,u5
  Cl_delta_ail : Interpolation_n-D  Table=AeroCoeff.Cl_delta_ail  InternalRulePriority=Speed
  Cl_delta_ail_lef : Interpolation_n-D  Table=AeroCoeff.Cl_delta_ail_lef  InternalRulePriority=Speed
  Cl_delta_r : Interpolation_n-D  Table=AeroCoeff.Cl_delta_r  InternalRulePriority=Speed
  Cl_elevator0 : Interpolation_n-D  Table=AeroCoeff.Cl_elevator0
  Cl_lef : Interpolation_n-D  Table=AeroCoeff.Cl_lef  InternalRulePriority=Speed
  Cl_p : Interpolation_n-D  NumberOfTableDimensions=1  Table=AeroCoeff.Cl_p  InternalRulePriority=Speed
      settings: InputPortMap=u0,u1
  Cl_r : Interpolation_n-D  NumberOfTableDimensions=1  Table=AeroCoeff.Cl_r  InternalRulePriority=Speed
      settings: InputPortMap=u0,u1
  Gain : Gain  Gain=1/20
  Gain1 : Gain  Gain=1/30
  Product{,1,4..8} (7 alike) : Product
  Subtract : Sum  Inputs=+-
  Subtract1 : Sum  Inputs=+-
  Subtract2 : Sum  Inputs=+--
  Subtract3 : Sum  Inputs=+-
  Subtract5 : Sum
  Subtract6 : Sum
  Subtract7 : Sum
  Subtract8 : Sum  Inputs=+++++
  alpha Prelookup : PreLookup  BreakpointsData=AeroCoeff.alpha_prelookup  IndexSearchMethod=Linear search  BeginIndexSearchUsingPreviousIndexResult=on  DiagnosticForOutOfRangeInput=Warning
  beta Prelookup : PreLookup  BreakpointsData=AeroCoeff.beta_prelookup  IndexSearchMethod=Linear search  BeginIndexSearchUsingPreviousIndexResult=on  DiagnosticForOutOfRangeInput=Warning
  dCl_beta : Interpolation_n-D  NumberOfTableDimensions=1  Table=AeroCoeff.dCl_beta  InternalRulePriority=Speed
      settings: InputPortMap=u0,u1
  dCl_p_lef : Interpolation_n-D  NumberOfTableDimensions=1  Table=AeroCoeff.dCl_p_lef  InternalRulePriority=Speed
      settings: InputPortMap=u0,u1
  dCl_r_lef : Interpolation_n-D  NumberOfTableDimensions=1  Table=AeroCoeff.dCl_r_lef  InternalRulePriority=Speed
      settings: InputPortMap=u0,u1
  elevator Prelookup : PreLookup  BreakpointsData=AeroCoeff.elevator_prelookup1  IndexSearchMethod=Linear search  BeginIndexSearchUsingPreviousIndexResult=on  DiagnosticForOutOfRangeInput=Warning
  Cl_tot_hat : Outport  VectorParamsAs1DForOutWhenUnconnected=off
  gp_da1 : Outport  Port=2  VectorParamsAs1DForOutWhenUnconnected=off
  gp_dr1 : Outport  Port=3  VectorParamsAs1DForOutWhenUnconnected=off
  gr_da1 : Outport  Port=4  VectorParamsAs1DForOutWhenUnconnected=off
  gr_dr1 : Outport  Port=5  VectorParamsAs1DForOutWhenUnconnected=off
  wires:
  Cl_elevator0/1 -> Subtract3/2, Subtract1/2, Subtract/2
  beta Prelookup/1 -> Cl/3, Cl_lef/3, Cl_elevator0/3, Cl_delta_ail_lef/3, Cl_delta_r/3, Cl_delta_ail/3
  Cl_delta_r/1 -> Subtract3/1
  Cl_lef/1 -> Subtract2/2, Subtract/1
  Subtract/1 -> Product/1
  Product6/1 -> Subtract7/2
  alpha Prelookup/1 -> dCl_r_lef/1, dCl_p_lef/1, dCl_beta/1, Cl_p/1, Cl_r/1, Cl_delta_r/1, Cl_delta_ail_lef/1, Cl_delta_ail/1, Cl_elevator0/1, Cl/1, Cl_lef/1
  Cl_p/1 -> Subtract7/1
  beta (deg)/1 -> beta Prelookup/1, Product8/2
  Subtract2/1 -> Product1/1
  alpha Prelookup/2 -> Cl_r/2, dCl_r_lef/2, dCl_p_lef/2, dCl_beta/2, Cl_p/2, Cl_delta_r/2, Cl_delta_ail_lef/2, Cl_delta_ail/2, Cl/2, Cl_lef/2, Cl_elevator0/2
  alpha (deg)/1 -> alpha Prelookup/1
  Product/1 -> Subtract8/2
  Subtract6/1 -> Product5/2
  rb_2v/1 -> Product5/1
  Cl_delta_ail/1 -> Subtract1/1
  elevator Prelookup/1 -> Cl/5
  Product7/1 -> Subtract8/4
  Subtract7/1 -> Product7/1
  Product5/1 -> Subtract8/3
  dCl_r_lef/1 -> Product4/1
  Subtract3/1 -> Gain1/1
  Subtract1/1 -> Subtract2/3, Subtract5/1
  dlef/1 -> Product6/1, Product4/2, Product/2, Product1/2
  Cl_delta_ail_lef/1 -> Subtract2/1
  beta Prelookup/2 -> Cl/4, Cl_lef/4, Cl_elevator0/4, Cl_delta_ail/4, Cl_delta_ail_lef/4, Cl_delta_r/4
  Product4/1 -> Subtract6/2
  dCl_beta/1 -> Product8/1
  Product1/1 -> Subtract5/2
  dCl_p_lef/1 -> Product6/2
  Product8/1 -> Subtract8/5
  Cl_r/1 -> Subtract6/1
  elevator Prelookup/2 -> Cl/6
  Cl/1 -> Subtract8/1
  pb_2v/1 -> Product7/2
  elevator (deg)/1 -> elevator Prelookup/1
  Subtract8/1 -> Cl_tot_hat/1
  Subtract5/1 -> Gain/1
  Gain/1 -> gp_da1/1, gr_da1/1
  Gain1/1 -> gp_dr1/1, gr_dr1/1

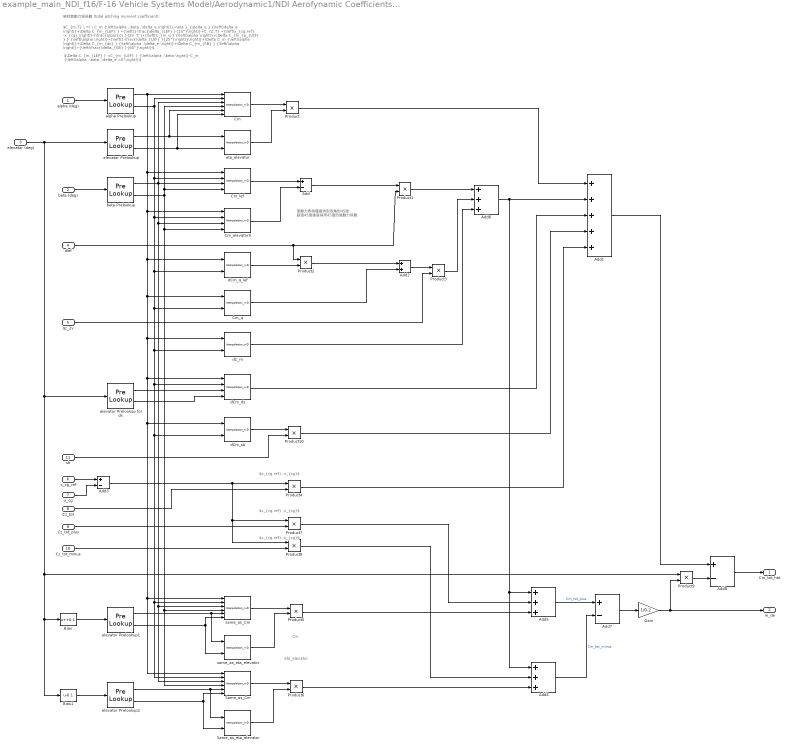
== system example_main_NDI_f16/F-16 Vehicle Systems Model/Aerodynamic1/NDI Aerofynamic Coefficients/CmT ==
  note: $x_{cg,ref} -x_{cg}$
  note: eta_elevator
  note: Cm
  note: 氣動力表格僅提供到攻角到45度，
      | 超過45度後皆採用45度的氣動力係數
  note: $x_{cg,ref} -x_{cg}$
  note: $x_{cg,ref} -x_{cg}$
  note: $C_{m,T} \ =\ \ C_m {\left(\alpha ,\beta ,\delta_e \right)}{∙\eta }_{\delta_e } {\left(\delta_e \right)}+\Delta C_{m_{LEF} } ∙{\left(1-\frac{\delta_{LEF} }{25°}\right)}+C_{Z,T} ∙{\left(x_{cg,ref} -x_{cg} \right)}+\frac{q\bar{c} }{2V_T }∙{\left[C_{m_q } {\left(\alpha \right)}+\Delta C_{m_{q_{LEF} } } {\left(\alpha \right)}∙{\left(1-\frac{\delta_{LEF} }{25°}\right)}\right]}+\Delta C_m {\left(\alpha \right)}+\Delta C_{m_{ds} } {\left(\alpha ,\delta_e \right)}+\Delta C_{m_{SB} } {\left(\alpha \right)}∙{\left(\frac{\delta_{SB} }{60°}\right)}$
  note: $\Delta C_{m_{LEF} } =C_{m_{LEF} } {\left(\alpha ,\beta \right)}-C_m {\left(\alpha ,\beta ,\delta_e =0°\right)}$
  note: 俯仰氣動力矩係數 (total pitching moment coefficient)：
  alpha (deg) : Inport
  beta (deg) : Inport  Port=2
  elevator (deg) : Inport  Port=3
  dlef : Inport  Port=4
  qc_2v : Inport  Port=5
  x_cg_ref : Inport  Port=6
  x_cg : Inport  Port=7
  Cz_tot : Inport  Port=8
  Cz_tot_plus : Inport  Port=9
  Cz_tot_minus : Inport  Port=10
  sb : Inport  Port=11
  Add{,3,7..8} (4 alike) : Sum  Inputs=+-
  Add1 : Sum  Inputs=+++++
  Add2 : Sum
  Add4 : Sum  Inputs=+++
  Add5 : Sum  Inputs=+++
  Add6 : Sum  Inputs=+++
  Bias : Bias  Bias=+0.1
  Bias1 : Bias  Bias=-0.1
  Cm : Interpolation_n-D  NumberOfTableDimensions=3  Table=AeroCoeff.Cm
      settings: InputPortMap=u0,u1,u2,u3,u4,u5
  Cm_elevator0 : Interpolation_n-D  Table=AeroCoeff.Cm_elevator0
  Cm_lef : Interpolation_n-D  Table=AeroCoeff.Cm_lef
  Cm_q : Interpolation_n-D  NumberOfTableDimensions=1  Table=AeroCoeff.Cm_q
      settings: InputPortMap=u0,u1
  Gain : Gain  Gain=1/0.2
  Product{,1..10} (11 alike) : Product
  Same_as_Cm : Interpolation_n-D  NumberOfTableDimensions=3  Table=AeroCoeff.Cm
      settings: InputPortMap=u0,u1,u2,u3,u4,u5
  Same_as_eta_elevator : Interpolation_n-D  NumberOfTableDimensions=1  Table=AeroCoeff.eta_elevator
      settings: InputPortMap=u0,u1
  alpha Prelookup : PreLookup  BreakpointsData=AeroCoeff.alpha_prelookup  IndexSearchMethod=Linear search  BeginIndexSearchUsingPreviousIndexResult=on  DiagnosticForOutOfRangeInput=Warning
  beta Prelookup : PreLookup  BreakpointsData=AeroCoeff.beta_prelookup  IndexSearchMethod=Linear search  BeginIndexSearchUsingPreviousIndexResult=on  DiagnosticForOutOfRangeInput=Warning
  dC_m : Interpolation_n-D  NumberOfTableDimensions=1  Table=AeroCoeff.dC_m
      settings: InputPortMap=u0,u1
  dCm_ds : Interpolation_n-D  Table=AeroCoeff.dCm_ds
  dCm_q_lef : Interpolation_n-D  NumberOfTableDimensions=1  Table=AeroCoeff.dCm_q_lef
      settings: InputPortMap=u0,u1
  dCm_sb : Interpolation_n-D  NumberOfTableDimensions=1  Table=AeroCoeff.dCm_sb
      settings: InputPortMap=u0,u1
  elevator Prelookup : PreLookup  BreakpointsData=AeroCoeff.elevator_prelookup2  IndexSearchMethod=Linear search  BeginIndexSearchUsingPreviousIndexResult=on  DiagnosticForOutOfRangeInput=Warning
  elevator Prelookup for ds : PreLookup  BreakpointsData=AeroCoeff.elevator_prelookup3  IndexSearchMethod=Linear search  BeginIndexSearchUsingPreviousIndexResult=on  DiagnosticForOutOfRangeInput=Warning
  elevator Prelookup1 : PreLookup  BreakpointsData=AeroCoeff.elevator_prelookup2  IndexSearchMethod=Linear search  BeginIndexSearchUsingPreviousIndexResult=on  DiagnosticForOutOfRangeInput=Warning
  elevator Prelookup2 : PreLookup  BreakpointsData=AeroCoeff.elevator_prelookup2  IndexSearchMethod=Linear search  BeginIndexSearchUsingPreviousIndexResult=on  DiagnosticForOutOfRangeInput=Warning
  eta_elevator : Interpolation_n-D  NumberOfTableDimensions=1  Table=AeroCoeff.eta_elevator
      settings: InputPortMap=u0,u1
  same_as_Cm : Interpolation_n-D  NumberOfTableDimensions=3  Table=AeroCoeff.Cm
      settings: InputPortMap=u0,u1,u2,u3,u4,u5
  same_as_eta_elevator : Interpolation_n-D  NumberOfTableDimensions=1  Table=AeroCoeff.eta_elevator
      settings: InputPortMap=u0,u1
  Cm_tot_hat : Outport  VectorParamsAs1DForOutWhenUnconnected=off
  m_de : Outport  Port=2  VectorParamsAs1DForOutWhenUnconnected=off
  wires:
  Cm/1 -> Product/1
  Cm_lef/1 -> Add/1
  Add3/1 -> Product8/1, Product7/1, Product4/1
  Product3/1 -> Add6/2
  alpha Prelookup/1 -> Same_as_Cm/1, same_as_Cm/1, dCm_sb/1, dCm_ds/1, dC_m/1, Cm_q/1, dCm_q_lef/1, Cm_elevator0/1, Cm_lef/1, Cm/1
  Cm_elevator0/1 -> Add/2
  elevator Prelookup/1 -> Cm/5, eta_elevator/1
  dC_m/1 -> Add6/3
  alpha Prelookup/2 -> Cm/2, Same_as_Cm/2, same_as_Cm/2, dCm_sb/2, dCm_ds/2, dC_m/2, Cm_q/2, dCm_q_lef/2, Cm_elevator0/2, Cm_lef/2
  dlef/1 -> Product2/1, Product1/2
  elevator Prelookup/2 -> Cm/6, eta_elevator/2
  elevator (deg)/1 -> elevator Prelookup/1, Bias1/1, Bias/1, Product9/1, elevator Prelookup for ds/1
  Product1/1 -> Add6/1
  eta_elevator/1 -> Product/2
  beta Prelookup/2 -> Same_as_Cm/4, same_as_Cm/4, Cm_elevator0/4, Cm/4, Cm_lef/4
  Product2/1 -> Add2/1
  Cm_q/1 -> Add2/2
  beta Prelookup/1 -> Cm/3, Same_as_Cm/3, same_as_Cm/3, Cm_elevator0/3, Cm_lef/3
  Product/1 -> Add1/1
  dCm_q_lef/1 -> Product2/2
  Add2/1 -> Product3/1
  Add/1 -> Product1/1
  qc_2v/1 -> Product3/2
  alpha (deg)/1 -> alpha Prelookup/1
  Product4/1 -> Add1/5
  beta (deg)/1 -> beta Prelookup/1
  x_cg/1 -> Add3/2
  Add1/1 -> Add8/1
  Cz_tot/1 -> Product4/2
  x_cg_ref/1 -> Add3/1
  Bias/1 -> elevator Prelookup1/1
  Bias1/1 -> elevator Prelookup2/1
  elevator Prelookup1/1 -> same_as_Cm/5, same_as_eta_elevator/1
  elevator Prelookup1/2 -> same_as_Cm/6, same_as_eta_elevator/2
  elevator Prelookup2/1 -> Same_as_eta_elevator/1, Same_as_Cm/5
  elevator Prelookup2/2 -> Same_as_Cm/6, Same_as_eta_elevator/2
  same_as_Cm/1 -> Product5/1
  same_as_eta_elevator/1 -> Product5/2
  Same_as_Cm/1 -> Product6/1
  Same_as_eta_elevator/1 -> Product6/2
  Product5/1 -> Add5/3
  Cz_tot_plus/1 -> Product7/2
  Cz_tot_minus/1 -> Product8/2
  Product7/1 -> Add5/2
  Product6/1 -> Add4/3
  Product8/1 -> Add4/2
  Add6/1 -> Add1/2, Add4/1, Add5/1
  Add5/1 -> Add7/1  "Cm_tot_plus"
  Add4/1 -> Add7/2  "Cm_tot_minus"
  Add7/1 -> Gain/1
  Gain/1 -> m_de/1, Product9/2
  Product9/1 -> Add8/2
  Add8/1 -> Cm_tot_hat/1
  sb/1 -> Product10/2
  dCm_sb/1 -> Product10/1
  Product10/1 -> Add1/4
  elevator Prelookup for ds/1 -> dCm_ds/3
  elevator Prelookup for ds/2 -> dCm_ds/4
  dCm_ds/1 -> Add1/3
